simulink model "drone_dynamics"  (R2020b)
settings: Solver=VariableStepAuto  StartTime=0.0  StopTime=10.0  FixedStep=0.0005  RelTol=1e-3
values from neighbouring files (symbols this model uses):
  A = 0.048 * g/(2 * pi * 7.4 * 12000 / 60)^2    (= 5.44350649507e-09)    [drone_param.m]
  d = 0.000000001    (= 1e-09)    [drone_param.m]
  dT_max = 19200 / 60 * 2 * pi    (= 2010.6192983)    [drone_param.m]
  f_accsensor_samplerate = 1000    [drone_param.m]
  f_gyrosensor_samplerate = 2000    [drone_param.m]
  f_magsensor_samplerate = 20    [drone_param.m]
  g = 9.80665    [drone_param.m]
  I_xx = 0.0075    [drone_param.m]
  I_yy = 0.0075    [drone_param.m]
  I_zz = 0.5    [drone_param.m]
  J_r = 0.0000005    (= 5e-07)    [drone_param.m]
  K_d_angle = 0    [drone_param.m]
  K_d_pitch = 2.0    (= 2)    [drone_param.m]
  K_d_roll = 2.0    (= 2)    [drone_param.m]
  K_d_yaw = 0.0    (= 0)    [drone_param.m]
  K_i_pitch = 2.0    (= 2)    [drone_param.m]
  K_i_roll = 2.0    (= 2)    [drone_param.m]
  K_i_yaw = 0.00    (= 0)    [drone_param.m]
  K_p_pitch = 10.0    (= 10)    [drone_param.m]
  K_p_roll = 10.0    (= 10)    [drone_param.m]
  K_p_throttle = -5.0    (= -5)    [drone_param.m]
  K_p_yaw = 0.0    (= 0)    [drone_param.m]
  l = 0.05    [drone_param.m]
  m = 0.15    [drone_param.m]
  pitch_init = 10.0/360 * 2 * pi    (= 0.174532925199)    [drone_param.m]
  roll_init = 10.0/360 * 2 * pi    (= 0.174532925199)    [drone_param.m]
  T_0 = 78490 / 60 * 2 * pi    (= 8219.45357934)    [drone_param.m]
  x_init = 0.0    (= 0)    [drone_param.m]
  y_init = 0.0    (= 0)    [drone_param.m]
  yaw_init = 0.0/360 * 2 * pi    (= 0)    [drone_param.m]
  z_init = 0.0    (= 0)    [drone_param.m]
libraries: simulink x3
settings Model: Creator=moe  LastModifiedBy=moe

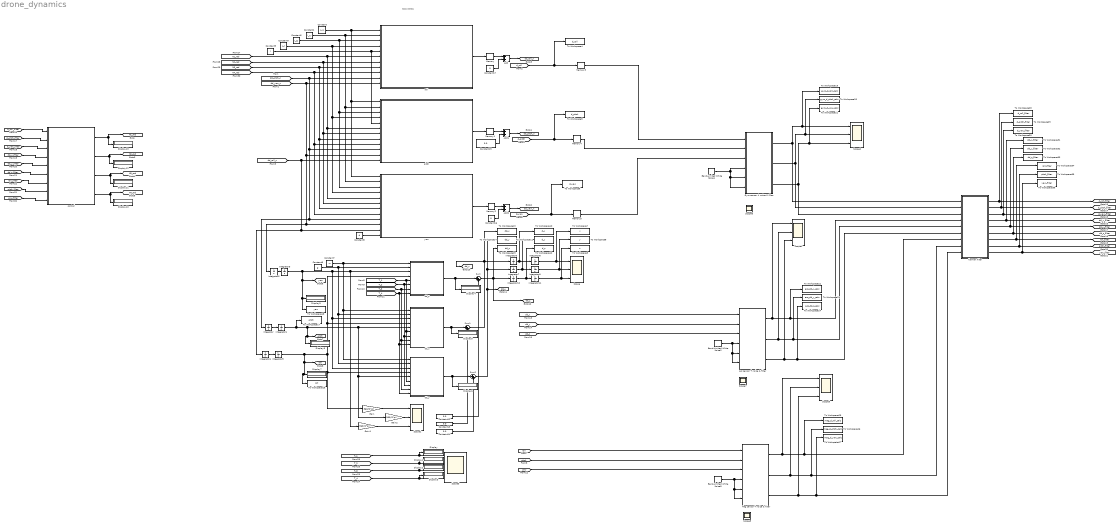
== system drone_dynamics ==
  note: 現実の物理系
  Acc sensor + noise & filter : Subsystem
  Add : Sum
  Add1 : Sum
  Add2 : Sum
  Band-Limited White Noise1 : simulink/Sources/Band-Limited White Noise  Cov=[0.00000003]  Ts=1/f_gyrosensor_samplerate  seed=[23341]
  Band-Limited White Noise2 : simulink/Sources/Band-Limited White Noise  Cov=[0.00000003]  Ts=1/f_accsensor_samplerate  seed=[1919]
  Band-Limited White Noise5 : simulink/Sources/Band-Limited White Noise  Cov=[0.00000003]  Ts=1/f_magsensor_samplerate  seed=[810]
  Constant : Constant  Value=I_xx
  Constant1 : Constant  Value=I_yy
  Constant{12..15} (4 alike) : Constant  Value=0.0
  Constant16 : Constant  Value=0
  Constant17 : Constant  Value=0
  Constant2 : Constant  Value=I_zz
  Constant3 : Constant  Value=d
  Constant4 : Constant  Value=J_r
  Constant5 : Constant  Value=l
  Constant7 : Constant  Value=m
  Constant8 : Constant  Value=g
  Display{,1..13} (14 alike) : Display
  Gain : Gain  Gain=360/(2*pi)
  Gain1 : Gain  Gain=360/(2*pi)
  Gain2 : Gain  Gain=360/(2*pi)
  Gyro sensor + noise & filter : Subsystem
  Integrator : Integrator  InitialCondition=pitch_init
  Integrator1 : Integrator  InitialCondition=pitch_init
  Integrator10 : Integrator  InitialCondition=z_init
  Integrator11 : Integrator  InitialCondition=z_init
  Integrator2 : Integrator  InitialCondition=yaw_init
  Integrator3 : Integrator  InitialCondition=yaw_init
  Integrator4 : Integrator  InitialCondition=roll_init
  Integrator5 : Integrator  InitialCondition=roll_init
  Integrator6 : Integrator  InitialCondition=x_init
  Integrator7 : Integrator  InitialCondition=y_init
  Integrator8 : Integrator  InitialCondition=x_init
  Integrator9 : Integrator  InitialCondition=y_init
  Karman filter : Subsystem
  Mag sensor + noise & filter : Subsystem
  Memory : Memory  InitialCondition=roll_init
  Memory1 : Memory  InitialCondition=pitch_init
  Memory2 : Memory  InitialCondition=yaw_init
  Memory3 : Memory  InitialCondition=roll_init
  Memory4 : Memory  InitialCondition=pitch_init
  Memory5 : Memory  InitialCondition=yaw_init
  Scope{,1..2,4..8} (8 alike) : Scope  NumInputPorts=3
  Scope3 : Scope  NumInputPorts=4
  Sum : Sum  Inputs=|++
  Sum1 : Sum  Inputs=|++
  Sum2 : Sum  Inputs=|++
  To Workspace10 : ToWorkspace  VariableName=d_x  SaveFormat=Timeseries  SampleTime=-1
  To Workspace11 : ToWorkspace  VariableName=d_y  SaveFormat=Timeseries  SampleTime=-1
  To Workspace12 : ToWorkspace  VariableName=d_z  SaveFormat=Timeseries  SampleTime=-1
  To Workspace13 : ToWorkspace  VariableName=dd_x  SaveFormat=Timeseries  SampleTime=-1
  To Workspace14 : ToWorkspace  VariableName=dd_y  SaveFormat=Timeseries  SampleTime=-1
  To Workspace15 : ToWorkspace  VariableName=dd_z  SaveFormat=Timeseries  SampleTime=-1
  To Workspace16 : ToWorkspace  VariableName=roll  SaveFormat=Timeseries  SampleTime=-1
  To Workspace17 : ToWorkspace  VariableName=pitch  SaveFormat=Timeseries  SampleTime=-1
  To Workspace18 : ToWorkspace  VariableName=yaw  SaveFormat=Timeseries  SampleTime=-1
  To Workspace19 : ToWorkspace  VariableName=gyro_d_roll_calc  SaveFormat=Timeseries  SampleTime=-1
  To Workspace20 : ToWorkspace  VariableName=gyro_d_pitch_calc  SaveFormat=Timeseries  SampleTime=-1
  To Workspace21 : ToWorkspace  VariableName=gyro_d_yaw_calc  SaveFormat=Timeseries  SampleTime=-1
  To Workspace22 : ToWorkspace  VariableName=acc_dd_x_calc  SaveFormat=Timeseries  SampleTime=-1
  To Workspace23 : ToWorkspace  VariableName=acc_dd_y_calc  SaveFormat=Timeseries  SampleTime=-1
  To Workspace24 : ToWorkspace  VariableName=acc_dd_z_calc  SaveFormat=Timeseries  SampleTime=-1
  To Workspace25 : ToWorkspace  VariableName=mag_d_roll_calc  SaveFormat=Timeseries  SampleTime=-1
  To Workspace26 : ToWorkspace  VariableName=mag_d_pitch_calc  SaveFormat=Timeseries  SampleTime=-1
  To Workspace27 : ToWorkspace  VariableName=mag_d_yaw_calc  SaveFormat=Timeseries  SampleTime=-1
  To Workspace28 : ToWorkspace  VariableName=d_roll_filter  SaveFormat=Timeseries  SampleTime=-1
  To Workspace29 : ToWorkspace  VariableName=d_pitch_filter  SaveFormat=Timeseries  SampleTime=-1
  To Workspace30 : ToWorkspace  VariableName=d_yaw_filter  SaveFormat=Timeseries  SampleTime=-1
  To Workspace31 : ToWorkspace  VariableName=dd_x_filter  SaveFormat=Timeseries  SampleTime=-1
  To Workspace32 : ToWorkspace  VariableName=dd_y_filter  SaveFormat=Timeseries  SampleTime=-1
  To Workspace33 : ToWorkspace  VariableName=dd_z_filter  SaveFormat=Timeseries  SampleTime=-1
  To Workspace34 : ToWorkspace  VariableName=roll_filter  SaveFormat=Timeseries  SampleTime=-1
  To Workspace35 : ToWorkspace  VariableName=pitch_filter  SaveFormat=Timeseries  SampleTime=-1
  To Workspace36 : ToWorkspace  VariableName=yaw_filter  SaveFormat=Timeseries  SampleTime=-1
  To Workspace4 : ToWorkspace  VariableName=d_roll  SaveFormat=Timeseries  SampleTime=-1
  To Workspace5 : ToWorkspace  VariableName=d_pitch  SaveFormat=Timeseries  SampleTime=-1
  To Workspace6 : ToWorkspace  VariableName=d_yaw  SaveFormat=Timeseries  SampleTime=-1
  To Workspace7 : ToWorkspace  VariableName=x  SaveFormat=Timeseries  SampleTime=-1
  To Workspace8 : ToWorkspace  VariableName=y  SaveFormat=Timeseries  SampleTime=-1
  To Workspace9 : ToWorkspace  VariableName=z  SaveFormat=Timeseries  SampleTime=-1
  control : Subsystem
  dd_x : MATLAB Function  TreatAsAtomicUnit=on
  dd_y : MATLAB Function  TreatAsAtomicUnit=on
  dd_z : MATLAB Function  TreatAsAtomicUnit=on
  pitch : Subsystem
  roll : Subsystem
  yaw : Subsystem
  tag scope: N1_rad=global, N2_rad=global, N3_rad=global, N4_rad=global, d_pitch_filter=global, d_roll_filter=global, d_yaw_filter=global, dd_pitch_n=global, dd_roll_n=global, dd_x=global, dd_x_filter=global, dd_y=global, dd_y_filter=global, dd_yaw_n=global, dd_z=global, dd_z_filter=global, pitch=global, pitch_filter=global, roll=global, roll_filter=global, yaw=global, yaw_filter=global
  wires:
  Constant/1 -> yaw/1(I_xx), pitch/1(I_xx), roll/1(I_xx)
  Constant1/1 -> yaw/2(I_yy), pitch/2(I_yy), roll/2(I_yy)
  Constant2/1 -> yaw/3(I_zz), pitch/3(I_zz), roll/3(I_zz)
  Constant4/1 -> yaw/4(J_r), pitch/4(J_r), roll/4(J_r)
  Constant3/1 -> yaw/12(d)
  Constant5/1 -> pitch/5(l), roll/5(l)
  yaw/1("dd_yaw ") -> Memory2/1
  roll/1("dd_roll ") -> Memory/1
  [T_1] -> dd_y/6(T1), dd_x/6(T1), dd_z/5(T1)
  [T_2] -> dd_y/7(T2), dd_x/7(T2), dd_z/6(T2)
  [T_3] -> dd_y/8(T3), dd_x/8(T3), dd_z/7(T3)
  [T_4] -> dd_y/9(T4), dd_x/9(T4), dd_z/8(T4)
  pitch/1("dd_pitch ") -> Memory1/1
  Constant7/1 -> dd_y/1(m), dd_x/1(m), dd_z/1(m)
  Constant8/1 -> dd_y/2(g), dd_x/2(g), dd_z/2(g)
  Integrator/1 -> Integrator1/1
  Integrator1/1 -> To Workspace17/1, Display8/1, [pitch], Gain2/1, dd_y/5(pitch), dd_x/5(pitch)  "pitch"
  Integrator2/1 -> Integrator3/1
  Integrator3/1 -> dd_y/3(yaw), dd_x/3(yaw), Gain1/1, dd_z/3(yaw), [yaw], To Workspace18/1, Display9/1  "yaw"
  Integrator4/1 -> Integrator5/1
  Integrator5/1 -> To Workspace16/1, Display7/1, [roll], dd_z/4(roll), dd_x/4(roll), Gain/1, dd_y/4(roll)  "roll"
  Integrator6/1 -> To Workspace10/1, Integrator8/1
  Integrator7/1 -> To Workspace11/1, Integrator9/1
  Integrator8/1 -> Scope/1, To Workspace7/1  "x"
  Integrator9/1 -> Scope/2, To Workspace8/1  "y"
  Integrator10/1 -> To Workspace12/1, Integrator11/1
  Integrator11/1 -> To Workspace9/1, Scope/3  "z"
  [T_1] -> Scope3/1, Display/1  "T_1"
  [T_2] -> Display1/1, Scope3/2  "T_2"
  [T_4] -> Display3/1, Scope3/4  "T_4"
  [T_3] -> Display2/1, Scope3/3  "T_3"
  [N1_rad] -> yaw/5(N1_rad), pitch/6(N1_rad), roll/6(N1_rad)
  [N2_rad] -> yaw/6(N2_rad), pitch/7(N2_rad), roll/7(N2_rad)
  [N3_rad] -> yaw/7(N3_rad), pitch/8(N3_rad), roll/8(N3_rad)
  [N4_rad] -> yaw/8(N4_rad), pitch/9(N4_rad), roll/9(N4_rad)
  [d_roll] -> To Workspace4/1, Memory3/1
  [d_pitch] -> To Workspace5/1, Memory4/1
  [d_yaw] -> To Workspace6/1, Memory5/1
  [roll] -> Mag sensor + noise & filter/1(roll_true)
  [pitch] -> Mag sensor + noise & filter/2(pitch_true)
  [yaw] -> Mag sensor + noise & filter/3(yaw_true)
  [dd_x] -> Acc sensor + noise & filter/1(dd_x_true)
  [dd_y] -> Acc sensor + noise & filter/2(dd_y_true)
  [dd_z] -> Acc sensor + noise & filter/3(dd_z_true)
  Acc sensor + noise & filter/1(dd_x_calc) -> Scope4/1, To Workspace22/1, Karman filter/4(dd_x_calc)
  Acc sensor + noise & filter/2(dd_y_calc) -> Scope4/2, To Workspace23/1, Karman filter/5(dd_y_calc)
  Acc sensor + noise & filter/3(dd_z_calc) -> To Workspace24/1, Karman filter/6(dd_z_calc), Scope4/3
  Mag sensor + noise & filter/1(roll_calc) -> Scope5/1, To Workspace25/1, Karman filter/7(roll_calc)
  Mag sensor + noise & filter/2(pitch_calc) -> Scope5/2, To Workspace26/1, Karman filter/8(pitch_calc)
  Mag sensor + noise & filter/3(yaw_calc) -> To Workspace27/1, Karman filter/9(yaw_calc), Scope5/3
  [d_roll_filter] -> control/1(d_roll_filter)
  [d_pitch_filter] -> control/2(d_pitch_filter)
  [d_yaw_filter] -> control/3(d_yaw_filter)
  [dd_x_filter] -> control/4(dd_x_filter)
  [dd_y_filter] -> control/5(dd_y_filter)
  [dd_z_filter] -> control/6(dd_z_filter)
  [roll_filter] -> control/7(roll_filter)
  [pitch_filter] -> control/8(pitch_filter)
  control/1(N1_rad) -> [N1_rad], Display13/1
  control/2(N2_rad) -> [N2_rad], Display12/1
  control/3(N3_rad) -> [N3_rad], Display11/1
  control/4(N4_rad) -> [N4_rad], Display10/1
  Memory3/1 -> Gyro sensor + noise & filter/1(d_roll_true)  "roll"
  Memory4/1 -> Gyro sensor + noise & filter/2(d_pitch_true)
  Memory5/1 -> Gyro sensor + noise & filter/3(d_yaw_true)
  dd_z/1(dd_z) -> Display4/1, Sum/1  "ddz"
  Sum/1 -> To Workspace15/1, [dd_z], Integrator10/1
  Constant12/1 -> Sum/2
  dd_x/1(dd_x) -> Display5/1, Sum1/1  "ddx"
  Sum1/1 -> To Workspace13/1, Integrator6/1, [dd_x]
  Constant13/1 -> Sum1/2
  dd_y/1(dd_y) -> Display6/1, Sum2/1  "ddy"
  Sum2/1 -> [dd_y], To Workspace14/1, Integrator7/1
  Constant14/1 -> Sum2/2
  [dd_yaw_n] -> Integrator2/1, yaw/10(dd_yaw), pitch/11(dd_yaw), roll/11(dd_yaw)
  [dd_pitch_n] -> Integrator/1, yaw/9(dd_pitch), pitch/10(dd_pitch), roll/10(dd_pitch)
  [dd_roll_n] -> Integrator4/1, yaw/11(dd_roll), pitch/12(dd_roll)
  Add/1 -> [dd_roll_n]
  Memory/1 -> Add/1  "roll"
  Add1/1 -> [dd_pitch_n]
  Memory1/1 -> Add1/1
  Memory2/1 -> Add2/1
  Add2/1 -> [dd_yaw_n]
  Constant15/1 -> Add1/2
  Constant16/1 -> Add2/2
  Constant17/1 -> Add/2
  Gain/1 -> Scope1/1  "roll"
  Gain1/1 -> Scope1/3  "yaw"
  Gain2/1 -> Scope1/2  "pitch"
  [yaw_filter] -> control/9(yaw_filter)
  Karman filter/1(d_roll_filter) -> To Workspace28/1, [d_roll_filter]
  Karman filter/9(yaw_filter) -> To Workspace36/1, [yaw_filter]
  Karman filter/7(roll_filter) -> To Workspace34/1, [roll_filter]
  Karman filter/5(dd_y_filter) -> To Workspace32/1, [dd_y_filter]
  Karman filter/4(dd_x_filter) -> To Workspace31/1, [dd_x_filter]
  Karman filter/3(d_yaw_filter) -> To Workspace30/1, [d_yaw_filter]
  Karman filter/2(d_pitch_filter) -> To Workspace29/1, [d_pitch_filter]
  Karman filter/6(dd_z_filter) -> To Workspace33/1, [dd_z_filter]
  Karman filter/8(pitch_filter) -> To Workspace35/1, [pitch_filter]
  Gyro sensor + noise & filter/1(d_roll_calc) -> Karman filter/1(d_roll_calc), To Workspace19/1, Scope2/1  "d_roll"
  Gyro sensor + noise & filter/2(d_pitch_calc) -> To Workspace20/1, Scope2/2, Karman filter/2(d_pitch_calc)  "d_pitch"
  Gyro sensor + noise & filter/3(d_yaw_calc) -> To Workspace21/1, Scope2/3, Karman filter/3(d_yaw_calc)  "d_yaw"
  Band-Limited White Noise1/1 -> Gyro sensor + noise & filter/6(d_yaw_noise), Gyro sensor + noise & filter/5(d_pitch_noise), Gyro sensor + noise & filter/4(d_roll_noise)
  Band-Limited White Noise2/1 -> Acc sensor + noise & filter/6(dd_z_noise), Acc sensor + noise & filter/5(dd_y_noise), Acc sensor + noise & filter/4(dd_x_noise)
  Band-Limited White Noise5/1 -> Mag sensor + noise & filter/6(yaw_noise), Mag sensor + noise & filter/5(pitch_noise), Mag sensor + noise & filter/4(roll_noise)

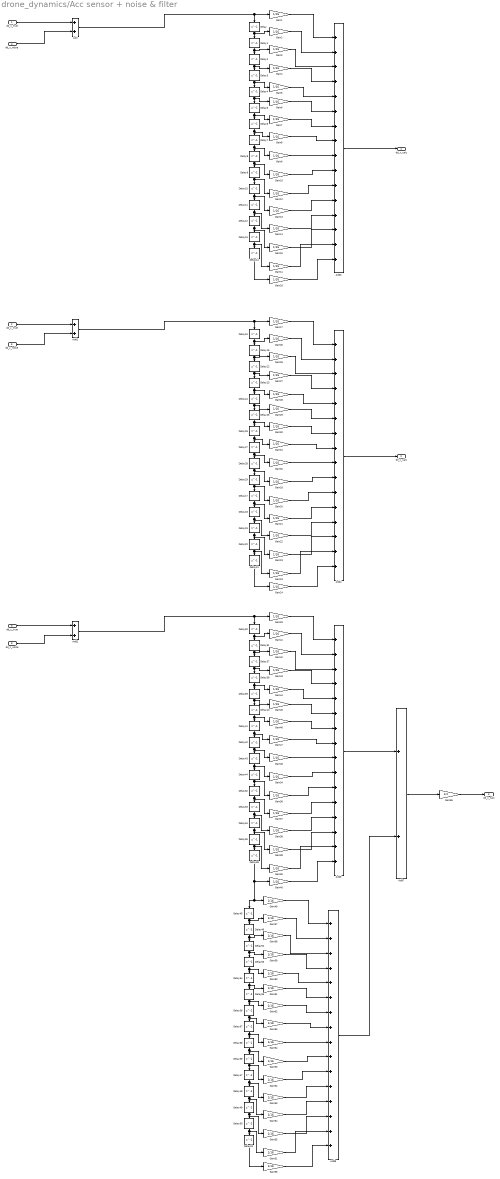
== system drone_dynamics/Acc sensor + noise & filter ==
  dd_x_true : Inport
  dd_y_true : Inport  Port=2
  dd_z_true : Inport  Port=3
  dd_x_noise : Inport  Port=4
  dd_y_noise : Inport  Port=5
  dd_z_noise : Inport  Port=6
  Add{,1..2,7} (4 alike) : Sum
  Add{3..6} (4 alike) : Sum  Inputs=++++++++++++++++
  Delay{,1..59} (60 alike) : Delay  DelayLength=1  InitialCondition=0
  Gain{1..64} (64 alike) : Gain  Gain=1/16
  Gain65 : Gain  Gain=1/2
  dd_x_calc : Outport
  dd_y_calc : Outport  Port=2
  dd_z_calc : Outport  Port=3
  wires:
  dd_x_true/1 -> Add/1
  dd_y_true/1 -> Add1/1
  dd_z_true/1 -> Add2/1
  dd_x_noise/1 -> Add/2
  dd_y_noise/1 -> Add1/2
  dd_z_noise/1 -> Add2/2
  Gain17/1 -> Add4/1
  Gain27/1 -> Add4/4
  Gain29/1 -> Add4/6
  Gain23/1 -> Add4/14
  Delay10/1 -> Gain13/1, Delay11/1
  Gain32/1 -> Add4/9
  Gain26/1 -> Add4/3
  Delay22/1 -> Gain27/1, Delay23/1
  Delay23/1 -> Gain28/1, Delay24/1
  Add4/1 -> dd_y_calc/1
  Gain14/1 -> Add3/13
  Gain11/1 -> Add3/15
  Gain8/1 -> Add3/8
  Gain10/1 -> Add3/10
  Gain12/1 -> Add3/11
  Gain2/1 -> Add3/2
  Add1/1 -> Delay15/1, Gain17/1
  Gain13/1 -> Add3/12
  Gain3/1 -> Add3/3
  Gain15/1 -> Add3/14
  Delay27/1 -> Gain32/1, Delay28/1
  Gain16/1 -> Add3/16
  Delay14/1 -> Gain16/1
  Gain34/1 -> Add5/10
  Gain47/1 -> Add5/8
  Gain33/1 -> Add5/1
  Gain43/1 -> Add5/4
  Gain46/1 -> Add5/7
  Gain48/1 -> Add5/9
  Gain42/1 -> Add5/3
  Gain37/1 -> Add5/12
  Gain9/1 -> Add3/9
  Gain7/1 -> Add3/7
  Gain35/1 -> Add5/15
  Gain6/1 -> Add3/6
  Gain44/1 -> Add5/5
  Gain31/1 -> Add4/8
  Add2/1 -> Delay30/1, Gain33/1
  Gain1/1 -> Add3/1
  Gain28/1 -> Add4/5
  Delay7/1 -> Gain9/1, Delay8/1
  Add3/1 -> dd_x_calc/1
  Delay3/1 -> Gain5/1, Delay4/1
  Delay2/1 -> Gain4/1, Delay3/1
  Delay1/1 -> Gain3/1, Delay2/1
  Delay/1 -> Gain2/1, Delay1/1
  Delay35/1 -> Gain35/1, Delay36/1
  Delay17/1 -> Gain21/1, Delay18/1
  Delay16/1 -> Gain26/1, Delay22/1
  Gain45/1 -> Add5/6
  Gain20/1 -> Add4/11
  Delay29/1 -> Gain20/1, Delay17/1
  Delay12/1 -> Gain15/1, Delay13/1
  Gain41/1 -> Add5/2
  Delay33/1 -> Gain38/1, Delay34/1
  Delay32/1 -> Gain37/1, Delay33/1
  Delay37/1 -> Gain43/1, Delay38/1
  Gain4/1 -> Add3/4
  Delay31/1 -> Gain42/1, Delay37/1
  Delay38/1 -> Gain44/1, Delay39/1
  Gain38/1 -> Add5/13
  Add/1 -> Delay/1, Gain1/1
  Delay43/1 -> Gain34/1, Delay44/1
  Gain36/1 -> Add5/11
  Delay42/1 -> Gain48/1, Delay43/1
  Gain19/1 -> Add4/15
  Gain21/1 -> Add4/12
  Delay41/1 -> Gain47/1, Delay42/1
  Delay39/1 -> Gain45/1, Delay40/1
  Delay40/1 -> Gain46/1, Delay41/1
  Delay9/1 -> Gain12/1, Delay10/1
  Delay11/1 -> Gain14/1, Delay12/1
  Delay6/1 -> Gain8/1, Delay7/1
  Delay25/1 -> Gain30/1, Delay26/1
  Gain18/1 -> Add4/10
  Gain5/1 -> Add3/5
  Delay5/1 -> Gain7/1, Delay6/1
  Gain25/1 -> Add4/2
  Gain22/1 -> Add4/13
  Delay28/1 -> Gain18/1, Delay29/1
  Delay19/1 -> Gain23/1, Delay20/1
  Gain30/1 -> Add4/7
  Delay21/1 -> Gain24/1
  Delay15/1 -> Gain25/1, Delay16/1
  Delay18/1 -> Gain22/1, Delay19/1
  Delay20/1 -> Gain19/1, Delay21/1
  Delay26/1 -> Gain31/1, Delay27/1
  Delay24/1 -> Gain29/1, Delay25/1
  Delay4/1 -> Gain6/1, Delay5/1
  Delay13/1 -> Gain11/1, Delay14/1
  Delay30/1 -> Gain41/1, Delay31/1
  Delay8/1 -> Gain10/1, Delay9/1
  Delay34/1 -> Gain39/1, Delay35/1
  Delay44/1 -> Gain36/1, Delay32/1
  Gain24/1 -> Add4/16
  Gain39/1 -> Add5/14
  Gain40/1 -> Add5/16
  Add5/1 -> Add7/1
  Add6/1 -> Add7/2
  Gain65/1 -> dd_z_calc/1
  Add7/1 -> Gain65/1
  Delay55/1 -> Gain62/1, Delay56/1
  Delay59/1 -> Gain52/1, Delay47/1
  Delay49/1 -> Gain55/1, Delay50/1
  Gain55/1 -> Add6/14
  Gain59/1 -> Add6/4
  Gain49/1 -> Add6/1
  Delay45/1 -> Gain57/1, Delay46/1
  Gain50/1 -> Add6/10
  Delay54/1 -> Gain61/1, Delay55/1
  Gain60/1 -> Add6/5
  Gain64/1 -> Add6/9
  Gain53/1 -> Add6/12
  Gain62/1 -> Add6/7
  Delay51/1 -> Gain56/1
  Gain56/1 -> Add6/16
  Delay50/1 -> Gain51/1, Delay51/1
  Gain58/1 -> Add6/3
  Delay56/1 -> Gain63/1, Delay57/1
  Delay53/1 -> Gain60/1, Delay54/1
  Gain54/1 -> Add6/13
  Delay46/1 -> Gain58/1, Delay52/1
  Delay52/1 -> Gain59/1, Delay53/1
  Delay48/1 -> Gain54/1, Delay49/1
  Delay36/1 -> Delay45/1, Gain49/1, Gain40/1
  Gain51/1 -> Add6/15
  Gain63/1 -> Add6/8
  Gain52/1 -> Add6/11
  Delay58/1 -> Gain50/1, Delay59/1
  Delay57/1 -> Gain64/1, Delay58/1
  Gain57/1 -> Add6/2
  Delay47/1 -> Gain53/1, Delay48/1
  Gain61/1 -> Add6/6

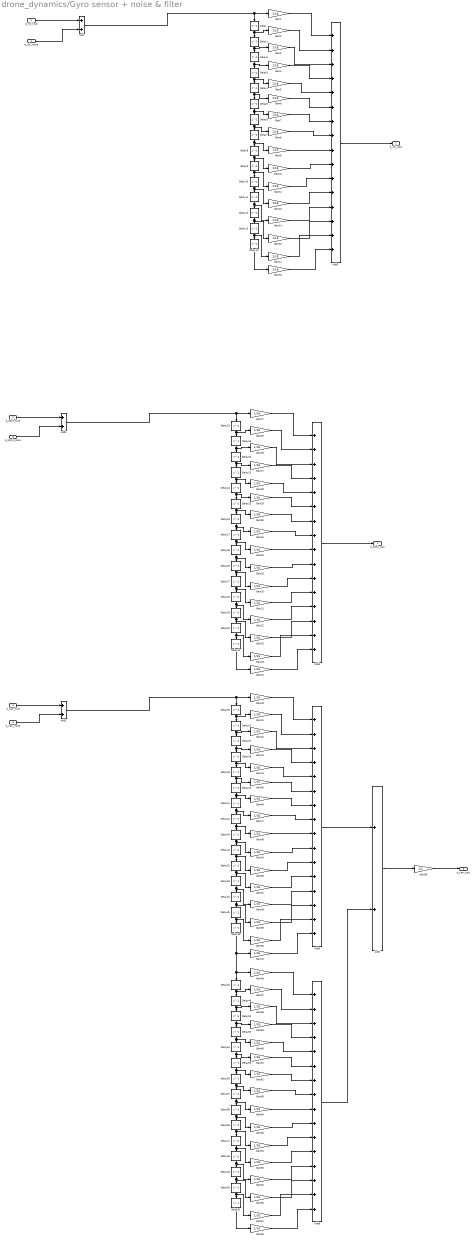
== system drone_dynamics/Gyro sensor + noise & filter ==
  d_roll_true : Inport
  d_pitch_true : Inport  Port=2
  d_yaw_true : Inport  Port=3
  d_roll_noise : Inport  Port=4
  d_pitch_noise : Inport  Port=5
  d_yaw_noise : Inport  Port=6
  Add{,1..2,7} (4 alike) : Sum
  Add{3..6} (4 alike) : Sum  Inputs=++++++++++++++++
  Delay{,1..59} (60 alike) : Delay  DelayLength=1  InitialCondition=0
  Gain{1..64} (64 alike) : Gain  Gain=1/16
  Gain65 : Gain  Gain=1/2
  d_roll_calc : Outport
  d_pitch_calc : Outport  Port=2
  d_yaw_calc : Outport  Port=3
  wires:
  d_roll_true/1 -> Add/1
  d_roll_noise/1 -> Add/2
  d_pitch_true/1 -> Add1/1
  d_yaw_true/1 -> Add2/1
  Delay/1 -> Gain2/1, Delay1/1
  Delay2/1 -> Gain4/1, Delay3/1
  Delay1/1 -> Gain3/1, Delay2/1
  Delay3/1 -> Gain5/1, Delay4/1
  Gain1/1 -> Add3/1
  Delay4/1 -> Gain6/1, Delay5/1
  Delay5/1 -> Gain7/1, Delay6/1
  Delay7/1 -> Gain9/1, Delay8/1
  Delay12/1 -> Gain15/1, Delay13/1
  Delay8/1 -> Gain10/1, Delay9/1
  Delay11/1 -> Gain14/1, Delay12/1
  Delay9/1 -> Gain12/1, Delay10/1
  Delay10/1 -> Gain13/1, Delay11/1
  Delay6/1 -> Gain8/1, Delay7/1
  Delay13/1 -> Gain11/1, Delay14/1
  Delay14/1 -> Gain16/1
  Gain2/1 -> Add3/2
  Gain3/1 -> Add3/3
  Gain4/1 -> Add3/4
  Gain5/1 -> Add3/5
  Gain6/1 -> Add3/6
  Gain7/1 -> Add3/7
  Gain8/1 -> Add3/8
  Gain9/1 -> Add3/9
  Gain10/1 -> Add3/10
  Gain12/1 -> Add3/11
  Gain13/1 -> Add3/12
  Gain14/1 -> Add3/13
  Gain15/1 -> Add3/14
  Gain11/1 -> Add3/15
  Gain16/1 -> Add3/16
  Add3/1 -> d_roll_calc/1
  Add/1 -> Delay/1, Gain1/1
  Gain31/1 -> Add4/8
  Gain18/1 -> Add4/10
  Gain28/1 -> Add4/5
  Gain19/1 -> Add4/15
  Gain25/1 -> Add4/2
  Gain21/1 -> Add4/12
  Gain26/1 -> Add4/3
  Delay21/1 -> Gain24/1
  Gain32/1 -> Add4/9
  Gain23/1 -> Add4/14
  Gain30/1 -> Add4/7
  Gain29/1 -> Add4/6
  Gain27/1 -> Add4/4
  Gain17/1 -> Add4/1
  Add1/1 -> Delay15/1, Gain17/1
  Delay27/1 -> Gain32/1, Delay28/1
  Add4/1 -> d_pitch_calc/1
  Delay23/1 -> Gain28/1, Delay24/1
  Delay22/1 -> Gain27/1, Delay23/1
  Delay16/1 -> Gain26/1, Delay22/1
  Delay17/1 -> Gain21/1, Delay18/1
  Delay29/1 -> Gain20/1, Delay17/1
  Gain20/1 -> Add4/11
  Delay28/1 -> Gain18/1, Delay29/1
  Gain22/1 -> Add4/13
  Delay18/1 -> Gain22/1, Delay19/1
  Delay25/1 -> Gain30/1, Delay26/1
  Delay24/1 -> Gain29/1, Delay25/1
  Delay26/1 -> Gain31/1, Delay27/1
  Delay20/1 -> Gain19/1, Delay21/1
  Delay15/1 -> Gain25/1, Delay16/1
  Delay19/1 -> Gain23/1, Delay20/1
  Gain24/1 -> Add4/16
  Gain47/1 -> Add5/8
  Gain34/1 -> Add5/10
  Gain44/1 -> Add5/5
  Gain35/1 -> Add5/15
  Gain41/1 -> Add5/2
  Gain37/1 -> Add5/12
  Gain42/1 -> Add5/3
  Gain48/1 -> Add5/9
  Gain39/1 -> Add5/14
  Gain46/1 -> Add5/7
  Gain45/1 -> Add5/6
  Gain43/1 -> Add5/4
  Gain33/1 -> Add5/1
  Add2/1 -> Delay30/1, Gain33/1
  Delay42/1 -> Gain48/1, Delay43/1
  Delay38/1 -> Gain44/1, Delay39/1
  Delay37/1 -> Gain43/1, Delay38/1
  Delay31/1 -> Gain42/1, Delay37/1
  Delay32/1 -> Gain37/1, Delay33/1
  Delay44/1 -> Gain36/1, Delay32/1
  Gain36/1 -> Add5/11
  Delay43/1 -> Gain34/1, Delay44/1
  Gain38/1 -> Add5/13
  Delay33/1 -> Gain38/1, Delay34/1
  Delay40/1 -> Gain46/1, Delay41/1
  Delay39/1 -> Gain45/1, Delay40/1
  Delay41/1 -> Gain47/1, Delay42/1
  Delay35/1 -> Gain35/1, Delay36/1
  Delay30/1 -> Gain41/1, Delay31/1
  Delay34/1 -> Gain39/1, Delay35/1
  Gain40/1 -> Add5/16
  d_pitch_noise/1 -> Add1/2
  d_yaw_noise/1 -> Add2/2
  Gain63/1 -> Add6/8
  Gain59/1 -> Add6/4
  Gain61/1 -> Add6/6
  Gain58/1 -> Add6/3
  Gain53/1 -> Add6/12
  Gain62/1 -> Add6/7
  Gain57/1 -> Add6/2
  Gain51/1 -> Add6/15
  Gain50/1 -> Add6/10
  Gain60/1 -> Add6/5
  Delay36/1 -> Delay45/1, Gain49/1, Gain40/1
  Delay51/1 -> Gain56/1
  Delay47/1 -> Gain53/1, Delay48/1
  Delay53/1 -> Gain60/1, Delay54/1
  Delay46/1 -> Gain58/1, Delay52/1
  Gain54/1 -> Add6/13
  Delay58/1 -> Gain50/1, Delay59/1
  Delay52/1 -> Gain59/1, Delay53/1
  Gain52/1 -> Add6/11
  Delay57/1 -> Gain64/1, Delay58/1
  Delay56/1 -> Gain63/1, Delay57/1
  Delay48/1 -> Gain54/1, Delay49/1
  Delay54/1 -> Gain61/1, Delay55/1
  Delay45/1 -> Gain57/1, Delay46/1
  Delay50/1 -> Gain51/1, Delay51/1
  Delay49/1 -> Gain55/1, Delay50/1
  Delay59/1 -> Gain52/1, Delay47/1
  Gain64/1 -> Add6/9
  Delay55/1 -> Gain62/1, Delay56/1
  Gain55/1 -> Add6/14
  Gain56/1 -> Add6/16
  Gain49/1 -> Add6/1
  Add5/1 -> Add7/1
  Add6/1 -> Add7/2
  Add7/1 -> Gain65/1
  Gain65/1 -> d_yaw_calc/1

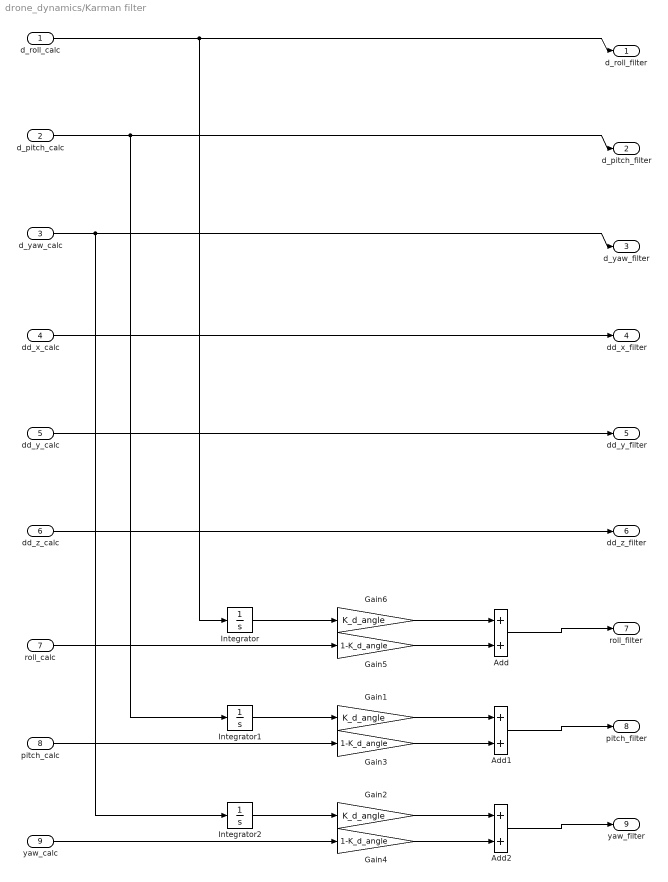
== system drone_dynamics/Karman filter ==
  d_roll_calc : Inport
  d_pitch_calc : Inport  Port=2
  d_yaw_calc : Inport  Port=3
  dd_x_calc : Inport  Port=4
  dd_y_calc : Inport  Port=5
  dd_z_calc : Inport  Port=6
  roll_calc : Inport  Port=7
  pitch_calc : Inport  Port=8
  yaw_calc : Inport  Port=9
  Add : Sum
  Add1 : Sum
  Add2 : Sum
  Gain1 : Gain  Gain=K_d_angle
  Gain2 : Gain  Gain=K_d_angle
  Gain3 : Gain  Gain=1-K_d_angle
  Gain4 : Gain  Gain=1-K_d_angle
  Gain5 : Gain  Gain=1-K_d_angle
  Gain6 : Gain  Gain=K_d_angle
  Integrator : Integrator  InitialCondition=roll_init
  Integrator1 : Integrator  InitialCondition=pitch_init
  Integrator2 : Integrator  InitialCondition=yaw_init
  d_roll_filter : Outport
  d_pitch_filter : Outport  Port=2
  d_yaw_filter : Outport  Port=3
  dd_x_filter : Outport  Port=4
  dd_y_filter : Outport  Port=5
  dd_z_filter : Outport  Port=6
  roll_filter : Outport  Port=7
  pitch_filter : Outport  Port=8
  yaw_filter : Outport  Port=9
  wires:
  dd_y_calc/1 -> dd_y_filter/1
  dd_x_calc/1 -> dd_x_filter/1
  dd_z_calc/1 -> dd_z_filter/1
  Gain3/1 -> Add1/2
  Gain4/1 -> Add2/2
  Gain2/1 -> Add2/1
  d_yaw_calc/1 -> Integrator2/1, d_yaw_filter/1
  Gain6/1 -> Add/1
  Gain5/1 -> Add/2
  Gain1/1 -> Add1/1
  d_roll_calc/1 -> Integrator/1, d_roll_filter/1
  d_pitch_calc/1 -> d_pitch_filter/1, Integrator1/1
  roll_calc/1 -> Gain5/1
  pitch_calc/1 -> Gain3/1
  yaw_calc/1 -> Gain4/1
  Add/1 -> roll_filter/1
  Add1/1 -> pitch_filter/1
  Add2/1 -> yaw_filter/1
  Integrator/1 -> Gain6/1
  Integrator1/1 -> Gain1/1
  Integrator2/1 -> Gain2/1

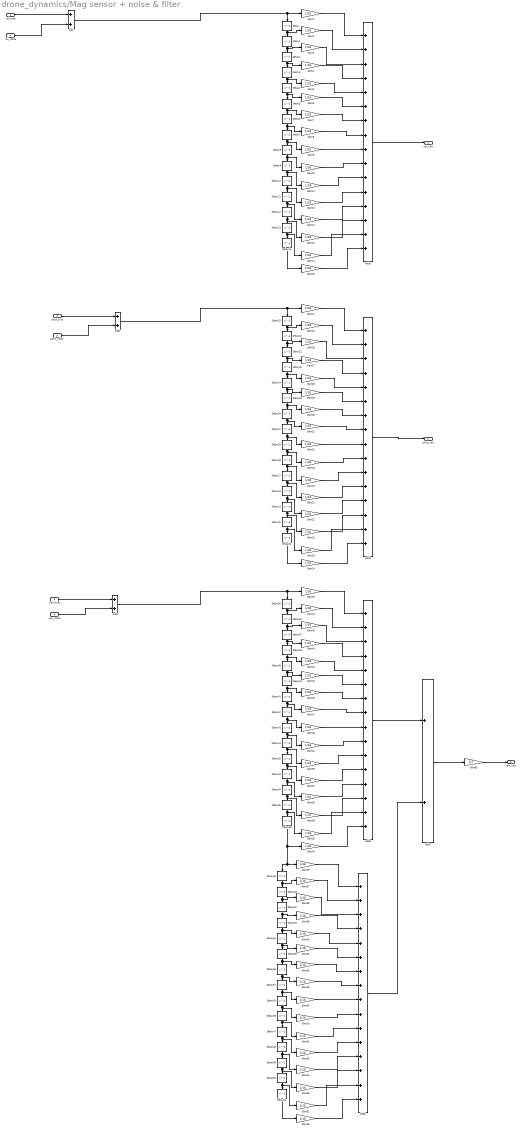
== system drone_dynamics/Mag sensor + noise & filter ==
  roll_true : Inport
  pitch_true : Inport  Port=2
  yaw_true : Inport  Port=3
  roll_noise : Inport  Port=4
  pitch_noise : Inport  Port=5
  yaw_noise : Inport  Port=6
  Add{,1..2,7} (4 alike) : Sum
  Add{3..6} (4 alike) : Sum  Inputs=++++++++++++++++
  Delay{,1..59} (60 alike) : Delay  DelayLength=1  InitialCondition=0
  Gain{1..64} (64 alike) : Gain  Gain=1/16
  Gain65 : Gain  Gain=1/2
  roll_calc : Outport
  pitch_calc : Outport  Port=2
  yaw_calc : Outport  Port=3
  wires:
  pitch_true/1 -> Add1/1
  yaw_true/1 -> Add2/1
  roll_true/1 -> Add/1
  roll_noise/1 -> Add/2
  pitch_noise/1 -> Add1/2
  yaw_noise/1 -> Add2/2
  Gain17/1 -> Add4/1
  Gain27/1 -> Add4/4
  Gain29/1 -> Add4/6
  Gain23/1 -> Add4/14
  Delay10/1 -> Gain13/1, Delay11/1
  Gain32/1 -> Add4/9
  Gain26/1 -> Add4/3
  Delay22/1 -> Gain27/1, Delay23/1
  Delay23/1 -> Gain28/1, Delay24/1
  Add4/1 -> pitch_calc/1
  Gain14/1 -> Add3/13
  Gain11/1 -> Add3/15
  Gain8/1 -> Add3/8
  Gain10/1 -> Add3/10
  Gain12/1 -> Add3/11
  Gain2/1 -> Add3/2
  Add1/1 -> Delay15/1, Gain17/1
  Gain13/1 -> Add3/12
  Gain3/1 -> Add3/3
  Gain15/1 -> Add3/14
  Delay27/1 -> Gain32/1, Delay28/1
  Gain16/1 -> Add3/16
  Delay14/1 -> Gain16/1
  Gain9/1 -> Add3/9
  Gain7/1 -> Add3/7
  Gain6/1 -> Add3/6
  Gain31/1 -> Add4/8
  Gain1/1 -> Add3/1
  Gain28/1 -> Add4/5
  Delay7/1 -> Gain9/1, Delay8/1
  Add3/1 -> roll_calc/1
  Delay3/1 -> Gain5/1, Delay4/1
  Delay2/1 -> Gain4/1, Delay3/1
  Delay1/1 -> Gain3/1, Delay2/1
  Delay/1 -> Gain2/1, Delay1/1
  Delay17/1 -> Gain21/1, Delay18/1
  Delay16/1 -> Gain26/1, Delay22/1
  Gain20/1 -> Add4/11
  Delay29/1 -> Gain20/1, Delay17/1
  Delay12/1 -> Gain15/1, Delay13/1
  Gain4/1 -> Add3/4
  Add/1 -> Delay/1, Gain1/1
  Gain19/1 -> Add4/15
  Gain21/1 -> Add4/12
  Delay9/1 -> Gain12/1, Delay10/1
  Delay11/1 -> Gain14/1, Delay12/1
  Delay6/1 -> Gain8/1, Delay7/1
  Delay25/1 -> Gain30/1, Delay26/1
  Gain18/1 -> Add4/10
  Gain5/1 -> Add3/5
  Delay5/1 -> Gain7/1, Delay6/1
  Gain25/1 -> Add4/2
  Gain22/1 -> Add4/13
  Delay28/1 -> Gain18/1, Delay29/1
  Delay19/1 -> Gain23/1, Delay20/1
  Gain30/1 -> Add4/7
  Delay21/1 -> Gain24/1
  Delay15/1 -> Gain25/1, Delay16/1
  Delay18/1 -> Gain22/1, Delay19/1
  Delay20/1 -> Gain19/1, Delay21/1
  Delay26/1 -> Gain31/1, Delay27/1
  Delay24/1 -> Gain29/1, Delay25/1
  Delay4/1 -> Gain6/1, Delay5/1
  Delay13/1 -> Gain11/1, Delay14/1
  Delay8/1 -> Gain10/1, Delay9/1
  Gain24/1 -> Add4/16
  Delay39/1 -> Gain45/1, Delay40/1
  Delay44/1 -> Gain36/1, Delay32/1
  Delay34/1 -> Gain39/1, Delay35/1
  Gain39/1 -> Add5/14
  Gain40/1 -> Add5/16
  Delay30/1 -> Gain41/1, Delay31/1
  Gain43/1 -> Add5/4
  Gain34/1 -> Add5/10
  Gain44/1 -> Add5/5
  Gain35/1 -> Add5/15
  Gain48/1 -> Add5/9
  Gain37/1 -> Add5/12
  Gain42/1 -> Add5/3
  Gain46/1 -> Add5/7
  Delay36/1 -> Delay45/1, Gain49/1, Gain40/1
  Gain54/1 -> Add6/13
  Delay46/1 -> Gain58/1, Delay52/1
  Gain58/1 -> Add6/3
  Delay56/1 -> Gain63/1, Delay57/1
  Gain56/1 -> Add6/16
  Add2/1 -> Delay30/1, Gain33/1
  Delay50/1 -> Gain51/1, Delay51/1
  Gain60/1 -> Add6/5
  Gain53/1 -> Add6/12
  Gain33/1 -> Add5/1
  Delay54/1 -> Gain61/1, Delay55/1
  Delay51/1 -> Gain56/1
  Gain62/1 -> Add6/7
  Gain49/1 -> Add6/1
  Delay49/1 -> Gain55/1, Delay50/1
  Gain59/1 -> Add6/4
  Gain55/1 -> Add6/14
  Gain50/1 -> Add6/10
  Delay45/1 -> Gain57/1, Delay46/1
  Delay55/1 -> Gain62/1, Delay56/1
  Gain51/1 -> Add6/15
  Delay48/1 -> Gain54/1, Delay49/1
  Delay52/1 -> Gain59/1, Delay53/1
  Add7/1 -> Gain65/1
  Gain64/1 -> Add6/9
  Gain57/1 -> Add6/2
  Gain52/1 -> Add6/11
  Gain61/1 -> Add6/6
  Delay57/1 -> Gain64/1, Delay58/1
  Delay58/1 -> Gain50/1, Delay59/1
  Add5/1 -> Add7/1
  Delay40/1 -> Gain46/1, Delay41/1
  Gain65/1 -> yaw_calc/1
  Delay35/1 -> Gain35/1, Delay36/1
  Delay47/1 -> Gain53/1, Delay48/1
  Delay41/1 -> Gain47/1, Delay42/1
  Delay38/1 -> Gain44/1, Delay39/1
  Gain38/1 -> Add5/13
  Gain63/1 -> Add6/8
  Delay31/1 -> Gain42/1, Delay37/1
  Delay53/1 -> Gain60/1, Delay54/1
  Delay37/1 -> Gain43/1, Delay38/1
  Delay59/1 -> Gain52/1, Delay47/1
  Add6/1 -> Add7/2
  Delay33/1 -> Gain38/1, Delay34/1
  Gain47/1 -> Add5/8
  Gain36/1 -> Add5/11
  Delay43/1 -> Gain34/1, Delay44/1
  Delay42/1 -> Gain48/1, Delay43/1
  Gain41/1 -> Add5/2
  Delay32/1 -> Gain37/1, Delay33/1
  Gain45/1 -> Add5/6

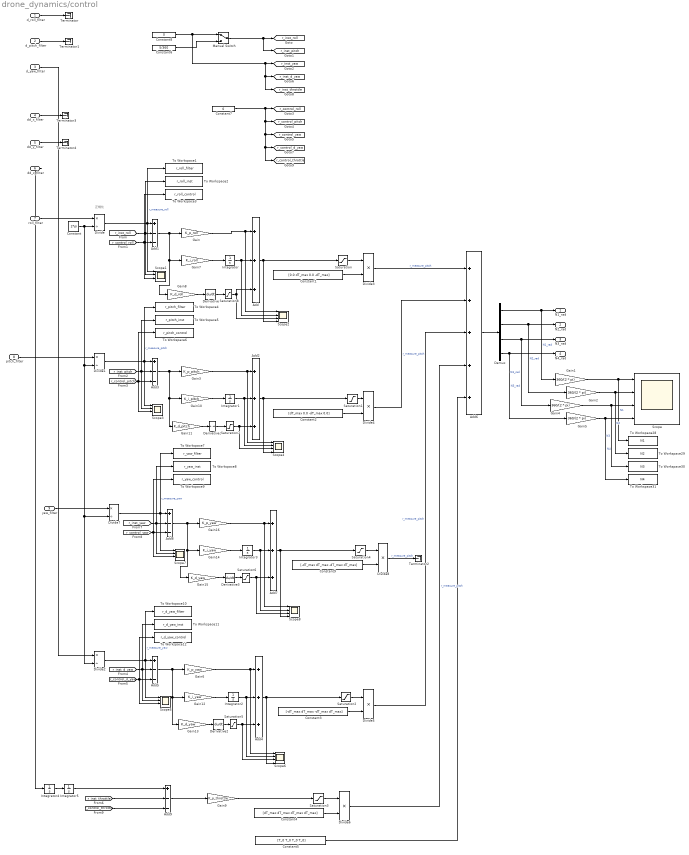
== system drone_dynamics/control ==
  note: 正規化
  d_roll_filter : Inport
  d_pitch_filter : Inport  Port=2
  d_yaw_filter : Inport  Port=3
  dd_x_filter : Inport  Port=4
  dd_y_filter : Inport  Port=5
  dd_z_filter : Inport  Port=6
  roll_filter : Inport  Port=7
  pitch_filter : Inport  Port=8
  yaw_filter : Inport  Port=9
  Add{,2,4,7} (4 alike) : Sum  Inputs=+++
  Add{1,3,5,8..9} (5 alike) : Sum  Inputs=+--
  Add6 : Sum  Inputs=+++++
  Constant : Constant  Value=2*pi
  Constant1 : Constant  Value=[0.0 dT_max 0.0 -dT_max]
  Constant2 : Constant  Value=[dT_max 0.0 -dT_max 0.0]
  Constant3 : Constant  Value=[-dT_max dT_max -dT_max dT_max]
  Constant4 : Constant  Value=[dT_max dT_max dT_max dT_max]
  Constant5 : Constant  Value=[T_0 T_0 T_0 T_0]
  Constant6 : Constant  Value=5/360
  Constant7 : Constant  Value=0
  Constant8 : Constant  Value=0
  Constant9 : Constant  Value=[-dT_max dT_max -dT_max dT_max]
  Demux : Demux
  Derivative{,1..3} (4 alike) : Derivative
  Divide{,1..2,7} (4 alike) : Product  Inputs=*/
  Divide{3..6,8} (5 alike) : Product  Inputs=**
  Gain : Gain  Gain=K_p_roll
  Gain{1..2,4..5} (4 alike) : Gain  Gain=360/(2 * pi)
  Gain10 : Gain  Gain=K_i_pitch
  Gain11 : Gain  Gain=K_d_pitch
  Gain12 : Gain  Gain=K_i_yaw
  Gain13 : Gain  Gain=K_d_yaw
  Gain14 : Gain  Gain=K_i_yaw
  Gain15 : Gain  Gain=K_d_yaw
  Gain16 : Gain  Gain=K_p_yaw
  Gain3 : Gain  Gain=K_p_pitch
  Gain6 : Gain  Gain=K_p_yaw
  Gain7 : Gain  Gain=K_i_roll
  Gain8 : Gain  Gain=K_d_roll
  Gain9 : Gain  Gain=K_p_throttle
  Integrator{,1..3} (4 alike) : Integrator
  Integrator4 : Integrator  InitialCondition=z_init
  Integrator5 : Integrator  InitialCondition=z_init
  Manual Switch : ManualSwitch
  Saturation{,1..8} (9 alike) : Saturate  UpperLimit=1  LowerLimit=-1
  Scope{,1..8} (9 alike) : Scope  NumInputPorts=4
  Terminator{,1..4} (5 alike) : Terminator
  To Workspace1 : ToWorkspace  VariableName=r_roll_filter  SaveFormat=Timeseries  SampleTime=-1
  To Workspace10 : ToWorkspace  VariableName=r_d_yaw_filter  SaveFormat=Timeseries  SampleTime=-1
  To Workspace11 : ToWorkspace  VariableName=r_d_yaw_inst  SaveFormat=Timeseries  SampleTime=-1
  To Workspace12 : ToWorkspace  VariableName=r_d_yaw_control  SaveFormat=Timeseries  SampleTime=-1
  To Workspace2 : ToWorkspace  VariableName=r_roll_inst  SaveFormat=Timeseries  SampleTime=-1
  To Workspace28 : ToWorkspace  VariableName=N1  SaveFormat=Timeseries  SampleTime=-1
  To Workspace29 : ToWorkspace  VariableName=N2  SaveFormat=Timeseries  SampleTime=-1
  To Workspace3 : ToWorkspace  VariableName=r_roll_control  SaveFormat=Timeseries  SampleTime=-1
  To Workspace30 : ToWorkspace  VariableName=N3  SaveFormat=Timeseries  SampleTime=-1
  To Workspace31 : ToWorkspace  VariableName=N4  SaveFormat=Timeseries  SampleTime=-1
  To Workspace4 : ToWorkspace  VariableName=r_pitch_filter  SaveFormat=Timeseries  SampleTime=-1
  To Workspace5 : ToWorkspace  VariableName=r_pitch_inst  SaveFormat=Timeseries  SampleTime=-1
  To Workspace6 : ToWorkspace  VariableName=r_pitch_control  SaveFormat=Timeseries  SampleTime=-1
  To Workspace7 : ToWorkspace  VariableName=r_yaw_filter  SaveFormat=Timeseries  SampleTime=-1
  To Workspace8 : ToWorkspace  VariableName=r_yaw_inst  SaveFormat=Timeseries  SampleTime=-1
  To Workspace9 : ToWorkspace  VariableName=r_yaw_control  SaveFormat=Timeseries  SampleTime=-1
  N1_rad : Outport
  N2_rad : Outport  Port=2
  N3_rad : Outport  Port=3
  N4_rad : Outport  Port=4
  tag scope: r_control_d_yaw=global, r_control_pitch=global, r_control_roll=global, r_control_throttle=global, r_control_yaw=global, r_inst_d_yaw=global, r_inst_pitch=global, r_inst_roll=global, r_inst_throttle=global, r_inst_yaw=global
  wires:
  d_roll_filter/1 -> Terminator/1
  d_pitch_filter/1 -> Terminator1/1
  dd_x_filter/1 -> Terminator3/1
  dd_y_filter/1 -> Terminator4/1
  dd_z_filter/1 -> Integrator4/1
  roll_filter/1 -> Divide/1
  pitch_filter/1 -> Divide1/1
  d_yaw_filter/1 -> Divide2/1
  Constant/1 -> Divide2/2, Divide7/2, Divide1/2, Divide/2
  Divide/1 -> To Workspace1/1, Scope1/1, Add1/1  "r_measure_roll"
  [r_inst_roll] -> To Workspace2/1, Scope1/2, Add1/2
  [r_control_roll] -> To Workspace3/1, Scope1/3, Add1/3
  Add1/1 -> Gain8/1, Gain7/1, Gain/1
  Gain7/1 -> Integrator/1
  Gain8/1 -> Derivative/1
  Derivative/1 -> Saturation8/1
  Integrator/1 -> Scope2/2, Add/2
  Gain/1 -> Scope2/1, Add/1
  [r_control_pitch] -> To Workspace6/1, Scope3/3, Add3/3
  Divide1/1 -> To Workspace4/1, Scope3/1, Add3/1  "r_measure_pitch"
  [r_inst_pitch] -> To Workspace5/1, Scope3/2, Add3/2
  Derivative1/1 -> Saturation7/1
  Add3/1 -> Gain11/1, Gain10/1, Gain3/1
  Gain10/1 -> Integrator1/1
  Gain3/1 -> Scope4/1, Add2/1
  Gain11/1 -> Derivative1/1
  Integrator1/1 -> Scope4/2, Add2/2
  Add5/1 -> Gain13/1, Gain12/1, Gain6/1
  Derivative2/1 -> Saturation5/1
  Gain12/1 -> Integrator2/1
  Gain6/1 -> Scope6/1, Add4/1
  [r_inst_d_yaw] -> To Workspace11/1, Scope5/2, Add5/2
  Gain13/1 -> Derivative2/1
  Integrator2/1 -> Scope6/2, Add4/2
  Divide2/1 -> To Workspace10/1, Scope5/1, Add5/1  "r_measure_yaw"
  [r_control_d_yaw] -> To Workspace12/1, Scope5/3, Add5/3
  Add/1 -> Scope2/4, Saturation/1
  Constant1/1 -> Divide3/2
  Add2/1 -> Scope4/4, Saturation1/1
  Constant2/1 -> Divide4/2
  Add4/1 -> Scope6/4, Saturation2/1
  Constant3/1 -> Divide5/2
  Divide3/1 -> Add6/1  "r_measure_pitch"
  Divide4/1 -> Add6/2  "r_measure_pitch"
  Constant4/1 -> Divide6/2
  Gain9/1 -> Saturation3/1
  Divide6/1 -> Add6/4  "r_measure_pitch"
  Constant5/1 -> Add6/5
  Add6/1 -> Demux/1
  Demux/1 -> Gain1/1, N1_rad/1  "N1_rad"
  Demux/2 -> Gain2/1, N2_rad/1  "N2_rad"
  Demux/3 -> Gain4/1, N3_rad/1  "N3_rad"
  Demux/4 -> Gain5/1, N4_rad/1  "N3_rad"
  Saturation/1 -> Divide3/1
  Saturation1/1 -> Divide4/1
  Saturation2/1 -> Divide5/1
  Saturation3/1 -> Divide6/1
  Constant7/1 -> [r_control_throttle], [r_control_d_yaw], [r_control_yaw], [r_control_pitch], [r_control_roll]
  Gain1/1 -> To Workspace28/1, Scope/1  "N1"
  Gain2/1 -> To Workspace29/1, Scope/2  "N2"
  Gain4/1 -> Scope/3, To Workspace30/1  "N3"
  Gain5/1 -> To Workspace31/1, Scope/4  "N4"
  Gain15/1 -> Derivative3/1
  Derivative3/1 -> Saturation6/1
  Saturation4/1 -> Divide8/1
  Gain14/1 -> Integrator3/1
  Gain16/1 -> Scope8/1, Add7/1
  Constant9/1 -> Divide8/2
  Add7/1 -> Scope8/4, Saturation4/1
  Divide7/1 -> To Workspace7/1, Scope7/1, Add8/1  "r_measure_yaw"
  [r_control_yaw] -> To Workspace9/1, Scope7/3, Add8/3
  Add8/1 -> Gain15/1, Gain14/1, Gain16/1
  [r_inst_yaw] -> To Workspace8/1, Scope7/2, Add8/2
  Integrator3/1 -> Scope8/2, Add7/2
  yaw_filter/1 -> Divide7/1
  Divide8/1 -> Terminator2/1  "r_measure_pitch"
  Divide5/1 -> Add6/3  "r_measure_pitch"
  Constant6/1 -> Manual Switch/2
  Constant8/1 -> [r_inst_throttle], [r_inst_d_yaw], [r_inst_yaw], Manual Switch/1
  Manual Switch/1 -> [r_inst_pitch], [r_inst_roll]
  Add9/1 -> Gain9/1
  [r_inst_throttle] -> Add9/2
  [r_control_throttle] -> Add9/3
  Integrator4/1 -> Integrator5/1
  Integrator5/1 -> Add9/1
  Saturation5/1 -> Scope6/3, Add4/3
  Saturation6/1 -> Scope8/3, Add7/3
  Saturation7/1 -> Scope4/3, Add2/3
  Saturation8/1 -> Scope2/3, Add/3

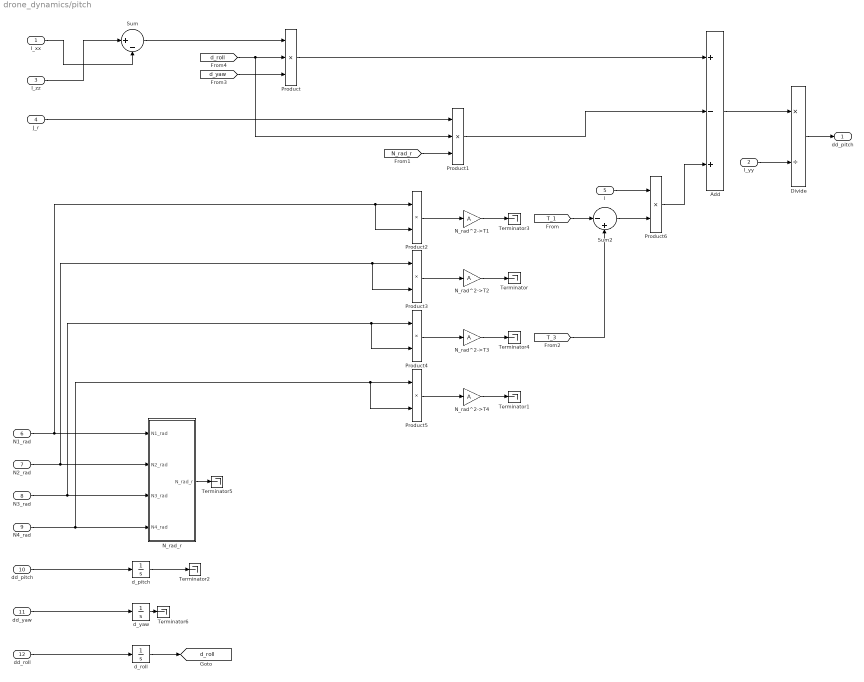
== system drone_dynamics/pitch ==
  I_xx : Inport
  I_yy : Inport  Port=2
  I_zz : Inport  Port=3
  J_r : Inport  Port=4
  l : Inport  Port=5
  N1_rad : Inport  Port=6
  N2_rad : Inport  Port=7
  N3_rad : Inport  Port=8
  N4_rad : Inport  Port=9
  dd_pitch : Inport  Port=10
  dd_yaw : Inport  Port=11
  dd_roll : Inport  Port=12
  Add : Sum  Inputs=+-+
  Divide : Product  Inputs=*/
  N_rad^2->T{1..4} (4 alike) : Gain  Gain=A
  N_rad_r : Subsystem
  Product : Product  Inputs=3
  Product1 : Product  Inputs=3
  Product{2..6} (5 alike) : Product
  Sum : Sum  Inputs=|+-
  Sum2 : Sum  Inputs=|-+
  Terminator{,1..6} (7 alike) : Terminator
  d_pitch : Integrator  InitialCondition=pitch_init
  d_roll : Integrator  InitialCondition=roll_init
  d_yaw : Integrator  InitialCondition=yaw_init
  "dd_pitch " : Outport
  tag scope: d_roll=global
  wires:
  N1_rad/1 -> Product2/2, Product2/1, N_rad_r/1(N1_rad)
  N2_rad/1 -> Product3/2, Product3/1, N_rad_r/2(N2_rad)
  N3_rad/1 -> Product4/2, Product4/1, N_rad_r/3(N3_rad)
  N4_rad/1 -> Product5/2, Product5/1, N_rad_r/4(N4_rad)
  Sum/1 -> Product/1
  dd_pitch/1 -> d_pitch/1
  dd_yaw/1 -> d_yaw/1
  Product/1 -> Add/1
  Product1/1 -> Add/2
  J_r/1 -> Product1/1
  Product2/1 -> N_rad^2->T1/1
  Product3/1 -> N_rad^2->T2/1
  Product4/1 -> N_rad^2->T3/1
  Product5/1 -> N_rad^2->T4/1
  Sum2/1 -> Product6/2
  l/1 -> Product6/1
  Product6/1 -> Add/3
  Divide/1 -> "dd_pitch "/1
  Add/1 -> Divide/1
  I_yy/1 -> Divide/2
  I_zz/1 -> Sum/1
  I_xx/1 -> Sum/2
  dd_roll/1 -> d_roll/1
  N_rad^2->T2/1 -> Terminator/1
  N_rad^2->T4/1 -> Terminator1/1
  d_pitch/1 -> Terminator2/1
  [T_1] -> Sum2/1
  [T_3] -> Sum2/2
  N_rad^2->T1/1 -> Terminator3/1
  N_rad^2->T3/1 -> Terminator4/1
  [N_rad_r] -> Product1/3
  N_rad_r/1(N_rad_r) -> Terminator5/1
  [d_yaw] -> Product/3
  [d_roll] -> Product1/2, Product/2
  d_roll/1 -> [d_roll]
  d_yaw/1 -> Terminator6/1

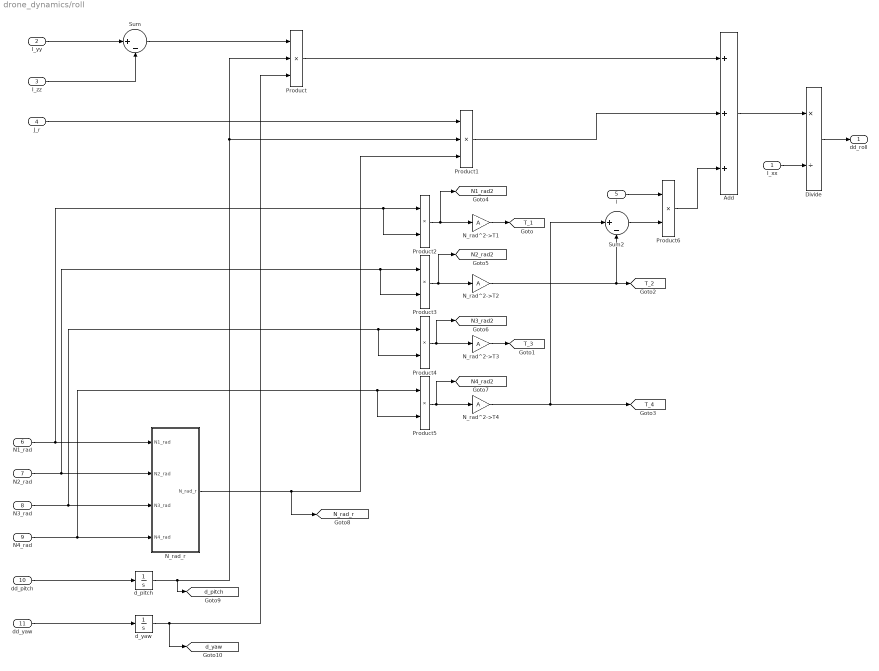
== system drone_dynamics/roll ==
  I_xx : Inport
  I_yy : Inport  Port=2
  I_zz : Inport  Port=3
  J_r : Inport  Port=4
  l : Inport  Port=5
  N1_rad : Inport  Port=6
  N2_rad : Inport  Port=7
  N3_rad : Inport  Port=8
  N4_rad : Inport  Port=9
  dd_pitch : Inport  Port=10
  dd_yaw : Inport  Port=11
  Add : Sum  Inputs=+++
  Divide : Product  Inputs=*/
  N_rad^2->T{1..4} (4 alike) : Gain  Gain=A
  N_rad_r : Subsystem
  Product : Product  Inputs=3
  Product1 : Product  Inputs=3
  Product{2..6} (5 alike) : Product
  Sum : Sum  Inputs=|+-
  Sum2 : Sum  Inputs=|+-
  d_pitch : Integrator  InitialCondition=pitch_init
  d_yaw : Integrator  InitialCondition=yaw_init
  "dd_roll " : Outport
  tag scope: N1_rad2=global, N2_rad2=global, N3_rad2=global, N4_rad2=global, N_rad_r=global, T_1=global, T_2=global, T_3=global, T_4=global, d_pitch=global, d_yaw=global
  wires:
  I_yy/1 -> Sum/1
  I_zz/1 -> Sum/2
  N1_rad/1 -> Product2/2, Product2/1, N_rad_r/1(N1_rad)
  N2_rad/1 -> Product3/2, Product3/1, N_rad_r/2(N2_rad)
  N3_rad/1 -> Product4/2, Product4/1, N_rad_r/3(N3_rad)
  N4_rad/1 -> Product5/2, Product5/1, N_rad_r/4(N4_rad)
  Sum/1 -> Product/1
  dd_pitch/1 -> d_pitch/1
  dd_yaw/1 -> d_yaw/1
  d_pitch/1 -> [d_pitch], Product1/2, Product/2
  d_yaw/1 -> [d_yaw], Product/3
  Product/1 -> Add/1
  Product1/1 -> Add/2
  J_r/1 -> Product1/1
  N_rad_r/1(N_rad_r) -> [N_rad_r], Product1/3
  Product2/1 -> [N1_rad2], N_rad^2->T1/1
  Product3/1 -> [N2_rad2], N_rad^2->T2/1
  Product4/1 -> [N3_rad2], N_rad^2->T3/1
  Product5/1 -> [N4_rad2], N_rad^2->T4/1
  N_rad^2->T4/1 -> [T_4], Sum2/1
  N_rad^2->T2/1 -> Sum2/2, [T_2]
  Sum2/1 -> Product6/2
  l/1 -> Product6/1
  Product6/1 -> Add/3
  N_rad^2->T1/1 -> [T_1]
  N_rad^2->T3/1 -> [T_3]
  Divide/1 -> "dd_roll "/1
  Add/1 -> Divide/1
  I_xx/1 -> Divide/2

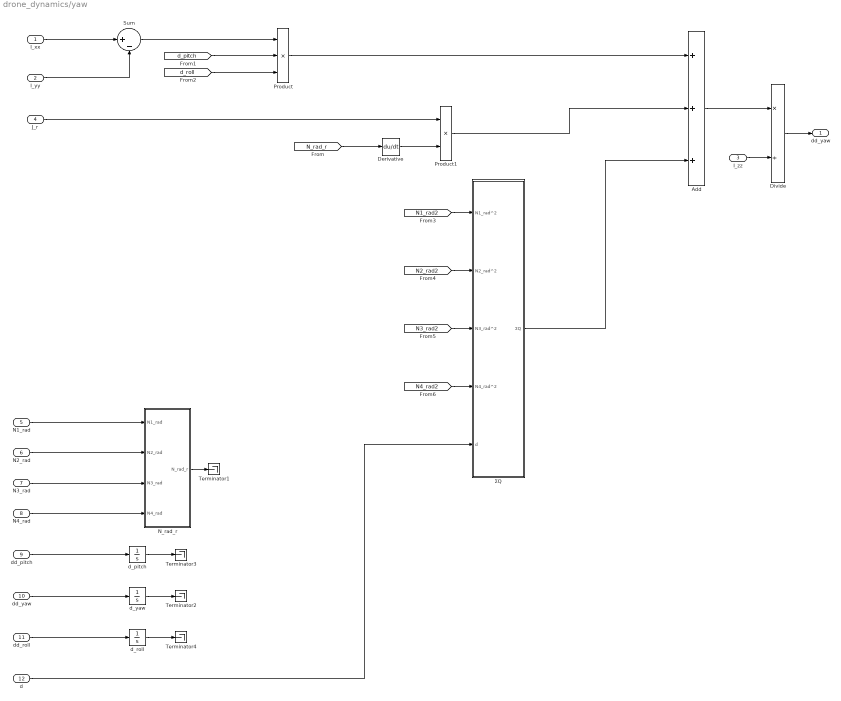
== system drone_dynamics/yaw ==
  I_xx : Inport
  I_yy : Inport  Port=2
  I_zz : Inport  Port=3
  J_r : Inport  Port=4
  N1_rad : Inport  Port=5
  N2_rad : Inport  Port=6
  N3_rad : Inport  Port=7
  N4_rad : Inport  Port=8
  dd_pitch : Inport  Port=9
  dd_yaw : Inport  Port=10
  dd_roll : Inport  Port=11
  d : Inport  Port=12
  Add : Sum  Inputs=+++
  Derivative : Derivative
  Divide : Product  Inputs=*/
  N_rad_r : Subsystem
  Product : Product  Inputs=3
  Product1 : Product
  Sum : Sum  Inputs=|+-
  Terminator{1..4} (4 alike) : Terminator
  d_pitch : Integrator  InitialCondition=pitch_init
  d_roll : Integrator  InitialCondition=roll_init
  d_yaw : Integrator  InitialCondition=yaw_init
  ΣQ : Subsystem
  "dd_yaw " : Outport
  wires:
  N1_rad/1 -> N_rad_r/1(N1_rad)
  N2_rad/1 -> N_rad_r/2(N2_rad)
  N3_rad/1 -> N_rad_r/3(N3_rad)
  N4_rad/1 -> N_rad_r/4(N4_rad)
  Sum/1 -> Product/1
  dd_pitch/1 -> d_pitch/1
  dd_yaw/1 -> d_yaw/1
  Product/1 -> Add/1
  Product1/1 -> Add/2
  J_r/1 -> Product1/1
  ΣQ/1(ΣQ) -> Add/3
  Divide/1 -> "dd_yaw "/1
  Add/1 -> Divide/1
  dd_roll/1 -> d_roll/1
  I_xx/1 -> Sum/1
  I_yy/1 -> Sum/2
  I_zz/1 -> Divide/2
  d_yaw/1 -> Terminator2/1
  Derivative/1 -> Product1/2
  d/1 -> ΣQ/5(d)
  [N_rad_r] -> Derivative/1
  [d_pitch] -> Product/2
  [d_roll] -> Product/3
  [N1_rad2] -> ΣQ/1(N1_rad^2)
  [N4_rad2] -> ΣQ/4(N4_rad^2)
  [N2_rad2] -> ΣQ/2(N2_rad^2)
  [N3_rad2] -> ΣQ/3(N3_rad^2)
  d_roll/1 -> Terminator4/1
  d_pitch/1 -> Terminator3/1
  N_rad_r/1(N_rad_r) -> Terminator1/1

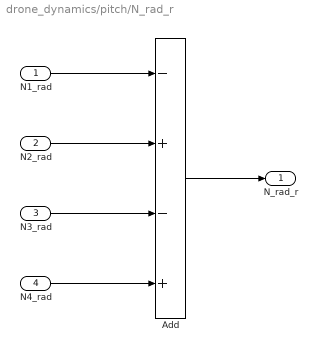
== system drone_dynamics/pitch/N_rad_r ==
  N1_rad : Inport
  N2_rad : Inport  Port=2
  N3_rad : Inport  Port=3
  N4_rad : Inport  Port=4
  Add : Sum  Inputs=-+-+
  N_rad_r : Outport
  wires:
  N1_rad/1 -> Add/1
  N2_rad/1 -> Add/2
  N3_rad/1 -> Add/3
  N4_rad/1 -> Add/4
  Add/1 -> N_rad_r/1

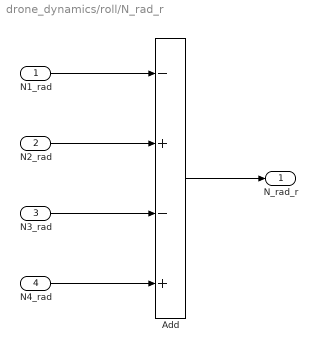
== system drone_dynamics/roll/N_rad_r ==
  N1_rad : Inport
  N2_rad : Inport  Port=2
  N3_rad : Inport  Port=3
  N4_rad : Inport  Port=4
  Add : Sum  Inputs=-+-+
  N_rad_r : Outport
  wires:
  N1_rad/1 -> Add/1
  N2_rad/1 -> Add/2
  N3_rad/1 -> Add/3
  N4_rad/1 -> Add/4
  Add/1 -> N_rad_r/1

== system drone_dynamics/yaw/N_rad_r ==
  N1_rad : Inport
  N2_rad : Inport  Port=2
  N3_rad : Inport  Port=3
  N4_rad : Inport  Port=4
  Add : Sum  Inputs=-+-+
  N_rad_r : Outport
  wires:
  N1_rad/1 -> Add/1
  N2_rad/1 -> Add/2
  N3_rad/1 -> Add/3
  N4_rad/1 -> Add/4
  Add/1 -> N_rad_r/1

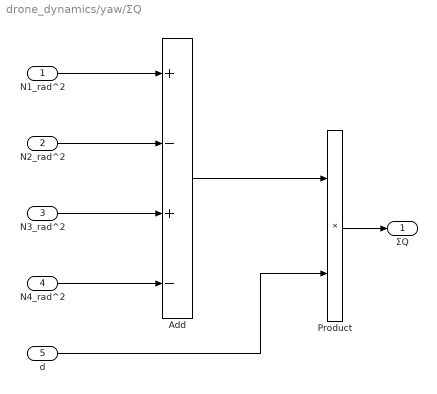
== system drone_dynamics/yaw/ΣQ ==
  N1_rad^2 : Inport
  N2_rad^2 : Inport  Port=2
  N3_rad^2 : Inport  Port=3
  N4_rad^2 : Inport  Port=4
  d : Inport  Port=5
  Add : Sum  Inputs=+-+-
  Product : Product
  ΣQ : Outport
  wires:
  N1_rad^2/1 -> Add/1
  N2_rad^2/1 -> Add/2
  N3_rad^2/1 -> Add/3
  N4_rad^2/1 -> Add/4
  Add/1 -> Product/1
  Product/1 -> ΣQ/1
  d/1 -> Product/2

== matlab function drone_dynamics/dd_x ==
  data: m input; dd_x output; g input; yaw input; roll input; pitch input; T1 input; T2 input; T3 input; T4 input
function dd_x = fcn(m, g, yaw, roll, pitch, T1, T2, T3, T4)
    dd_x = (sin(yaw) * sin(roll) + cos(yaw) * sin(pitch) * cos(roll)) * (T1 + T2 + T3 + T4)/m

== matlab function drone_dynamics/dd_z ==
  data: m input; dd_z output; g input; yaw input; roll input; T1 input; T2 input; T3 input; T4 input
function dd_z = fcn(m, g, yaw, roll, T1, T2, T3, T4)
    dd_z = - g + cos(yaw) * cos(roll) * (T1 + T2 + T3 + T4)/m

== matlab function drone_dynamics/dd_y ==
  data: m input; dd_y output; g input; yaw input; roll input; pitch input; T1 input; T2 input; T3 input; T4 input
function dd_y = fcn(m, g, yaw, roll, pitch, T1, T2, T3, T4)
    dd_y = ( - cos(yaw) * sin(roll) + sin(yaw) * sin(pitch) * cos(roll)) * (T1 + T2 + T3 + T4)/m
